simulink model "SIR_PWS_model"  (R2020a)
settings: Solver=VariableStepAuto  StartTime=0.0  StopTime=tf  MaxStep=0.01  RelTol=1e-3
undefined symbols (not defined in the file): beta, delta, gamma, mu, x0
settings Model: Creator=ciro  LastModifiedBy=ciro

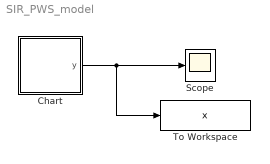
== system SIR_PWS_model ==
  Chart : Stateflow chart  TreatAsAtomicUnit=on
  Scope : Scope
  To Workspace : ToWorkspace  VariableName=x  SaveFormat=Timeseries  SampleTime=-1
  wires:
  Chart/1(y) -> To Workspace/1, Scope/1

== stateflow chart SIR_PWS_model/Chart ==
  settings: updateMethod=CONTINUOUS
  state initialState
  state f_zero
    during:
    x_dot = f_s;
    y = x;
  state f_plus
    during:
    x_dot = f_p;
    y = x;
  state f_minus
    during:
    x_dot = f_m;
    y=x;
  (default) -> initialState : {x = x0;}
  initialState -> f_plus [order 2] : [sigma > 0]
  initialState -> f_minus [order 1] : [sigma < 0]
  initialState -> f_zero [order 3] : [sigma == 0]
  f_zero -> f_minus [order 2] : [lie_p < 0 && lie_m < 0]
  f_zero -> f_plus [order 1] : [lie_p > 0 && lie_m > 0]
  f_plus -> f_zero [order 2] : [sigma <= 0 && lie_m > 0]
  f_minus -> f_zero [order 2] : [sigma >=0 && lie_p < 0 && lie_m > 0]
  f_plus -> f_minus [order 1] : [sigma <=0 && lie_m < 0]
  f_minus -> f_plus [order 1] : [sigma >= 0 && lie_p < 0 && lie_m < 0]
  data: f_s_val function_output; f_p_val function_output; f_m_val function_output; sigma_val function_output; lie_p_val function_output; lie_m_val function_output; y output; gamma parameter; mu parameter; delta parameter; beta parameter; x local; x0 parameter
  data x settings: updateMethod=SF_CONTINUOUS_TIME_DATA
  function f_s_val = f_s:
    | function f_s_val = f_s
    |     f_s_val = [mu-mu*x(1)-(gamma + mu)*delta; 0];
    | end
  function f_p_val = f_p:
    | function f_p_val = f_p
    |     f_p_val = [mu-mu*x(1); -(gamma+mu)*x(2)];
    | end
  function f_m_val = f_m:
    | function f_m_val = f_m
    |     f_m_val = [ mu-mu*x(1)-beta*x(1)*x(2);
    |         beta*x(1)*x(2)-(gamma+mu)*x(2)];
    | end
  function sigma_val = sigma:
    | function sigma_val = sigma
    |     sigma_val = x(2)-delta;
    | end
  function lie_p_val = lie_p:
    | function lie_p_val = lie_p
    |     lie_p_val = -(gamma+mu)*x(2);
    | end
  function lie_m_val = lie_m:
    | function lie_m_val = lie_m
    |     lie_m_val = beta*x(1)*x(2) -(gamma+mu)*x(2);
    | end
